simulink library "thc"  (R2021b)
settings: Solver=VariableStepAuto  StartTime=0.0  StopTime=10.0  RelTol=1e-3
undefined symbols (not defined in the file): ATHC_APTCQA_X_C, ATHC_APTCQB_X_C, ATHC_dAy_X_C, ATHC_Qeq_X_kmh, ATHC_VbaseC_X_C, ATHC_VbaseC_Y_W, ATHC_VbaseD_X_C, ATHC_VbaseH_X_C, FALSE, KTHC_ACMaxMinT_sec, KTHC_aDeice_K, KTHC_AGSDefLv_K, KTHC_AGSLv1_K, KTHC_AGSLv2_K, KTHC_AGSLv3_K, KTHC_AGSLv4_K, KTHC_AGSLv5_K, KTHC_AirIntUpdateT_sec, KTHC_APTCOneZoneMax_W, KTHC_APTCPeriod_cnt, KTHC_APTCPWMEN_flg, KTHC_APTCQMaxC_W, KTHC_APTCQminC_W, KTHC_APTCQminD_W, KTHC_APTCQminRe1_W, KTHC_APTCQminRe_W, KTHC_APTCQoffT_cnt, KTHC_APTCQonT_cnt, KTHC_APTCRiLeMaxDff_W, KTHC_APTCRiLeMinDff_W, KTHC_BatCoolT_cnt, KTHC_BatInTempDef_C, KTHC_bDeice_K, KTHC_CompMaxDeice_rpm, KTHC_CompMinDeice_rpm, KTHC_CompSotxvOp_K, KTHC_CompSotxvOpLow_rpm, KTHC_CompSpdmax_rpm, KTHC_CompSpdmaxBC1_rpm, KTHC_CompSpdmaxBC_rpm, KTHC_CompSpdmid1_rpm, KTHC_CompSpdmid2_rpm, KTHC_CompSpdmid3_rpm, KTHC_CompSpdmid_rpm, KTHC_CompSpdmin_rpm, KTHC_DAPTCQ1_W, KTHC_DAPTCQ2_W, KTHC_DAPTCQ3_W, KTHC_DcChSetTemp_C, KTHC_DehumidityEN_flg, KTHC_DeiceCycTime_K, KTHC_DriveLevelWPTCBAH1_W, KTHC_DriveLevelWPTCBAH2_W, KTHC_DriveLevelWPTCBAH3_W, KTHC_DriveLevelWPTCBAH4_W, KTHC_DriverSeatPos_flg, KTHC_DriveT1MinBAH_C, KTHC_DriveT2MaxBAH_C, KTHC_DriveT2MinBAH_C, KTHC_DriveT3MaxBAH_C ... (+379)
libraries: simulink x489
(part 10 of 17)

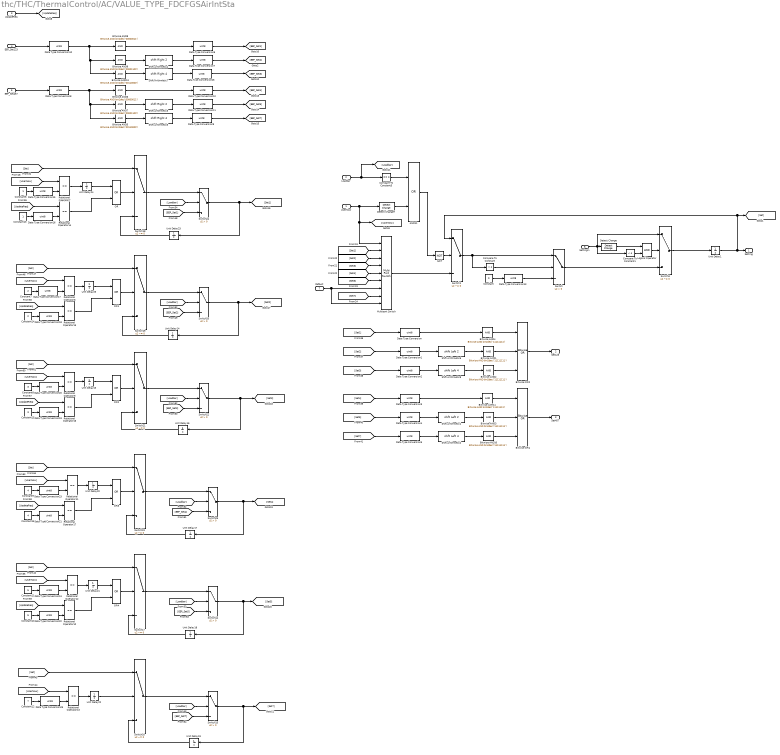
== system thc/THC/ThermalControl/AC/VALUE_TYPE_FDCFGSAirIntSta ==
  UserNow : Inport
  Loadbar : Inport  Port=2
  UpdateReq : Inport  Port=3
  EEP_Set123 : Inport  Port=4
  EEP_Set457 : Inport  Port=5
  SettingIn : Inport  Port=6
  Default : Inport  Port=7
  AND11 : Logic  Operator=OR  AllPortsSameDT=off  OutDataTypeStr=boolean
  Bitwise AND{1..4,10..11} (6 alike) : simulink/Logic and Bit Operations/Bitwise Operator  logicop=AND  UseBitMask=on  BitMask=bin2dec('11111111')  BitMaskRealWorld=Stored Integer
  Bitwise AND13 : simulink/Logic and Bit Operations/Bitwise Operator  logicop=AND  UseBitMask=on  BitMask=bin2dec('00110000')  BitMaskRealWorld=Stored Integer
  Bitwise AND5 : simulink/Logic and Bit Operations/Bitwise Operator  logicop=AND  UseBitMask=on  BitMask=bin2dec('00110000')  BitMaskRealWorld=Stored Integer
  Bitwise AND6 : simulink/Logic and Bit Operations/Bitwise Operator  logicop=AND  UseBitMask=on  BitMask=bin2dec('00000011')  BitMaskRealWorld=Stored Integer
  Bitwise AND7 : simulink/Logic and Bit Operations/Bitwise Operator  logicop=AND  UseBitMask=on  BitMask=bin2dec('00001100')  BitMaskRealWorld=Stored Integer
  Bitwise AND8 : simulink/Logic and Bit Operations/Bitwise Operator  logicop=AND  UseBitMask=on  BitMask=bin2dec('00000011')  BitMaskRealWorld=Stored Integer
  Bitwise AND9 : simulink/Logic and Bit Operations/Bitwise Operator  logicop=AND  UseBitMask=on  BitMask=bin2dec('00001100')  BitMaskRealWorld=Stored Integer
  Bitwise OR1 : simulink/Logic and Bit Operations/Bitwise Operator  logicop=OR  UseBitMask=off  NumInputPorts=3  BitMask=bin2dec('00000000000000000000')  BitMaskRealWorld=Stored Integer
  Bitwise OR2 : simulink/Logic and Bit Operations/Bitwise Operator  logicop=OR  UseBitMask=off  NumInputPorts=3  BitMask=bin2dec('00000000000000000000')  BitMaskRealWorld=Stored Integer
  Compare To Constant : simulink/Logic and Bit Operations/Compare To Constant  relop=<  const=4  OutDataTypeStr=boolean
  Compare To Constant1 : simulink/Logic and Bit Operations/Compare To Constant  relop=<  const=4  OutDataTypeStr=boolean
  Compare To Constant5 : simulink/Logic and Bit Operations/Compare To Constant  relop===  const=0  OutDataTypeStr=boolean
  Constant : Constant  Value=0
  Constant10 : Constant  Value=5  OutDataTypeStr=uint8
  Constant11 : Constant  Value=5  OutDataTypeStr=uint8
  Constant12 : Constant  Value=7  OutDataTypeStr=uint8
  Constant13 : Constant  OutDataTypeStr=uint8
  Constant14 : Constant  Value=2  OutDataTypeStr=uint8
  Constant15 : Constant  Value=3  OutDataTypeStr=uint8
  Constant16 : Constant  Value=4  OutDataTypeStr=uint8
  Constant6 : Constant  OutDataTypeStr=uint8
  Constant7 : Constant  Value=2  OutDataTypeStr=uint8
  Constant8 : Constant  Value=3  OutDataTypeStr=uint8
  Constant9 : Constant  Value=4  OutDataTypeStr=uint8
  Data Type Conversion{,1..13,15..26} (26 alike) : DataTypeConversion  OutDataTypeStr=uint8
  Detect Change : simulink/Logic and Bit Operations/Detect Change  vinit=0  OutDataTypeStr=boolean
  Detect Change7 : simulink/Logic and Bit Operations/Detect Change  vinit=0  OutDataTypeStr=boolean
  Logical Operator : Logic  AllPortsSameDT=off  OutDataTypeStr=boolean
  Multiport Switch : MultiPortSwitch  Inputs=7  DataPortForDefault=Additional data port  DiagnosticForDefault=None
  NOT : Logic  Operator=NOT  IconShape=distinctive  AllPortsSameDT=off  OutDataTypeStr=boolean
  OR{,1..4} (5 alike) : Logic  Operator=OR  AllPortsSameDT=off  OutDataTypeStr=boolean
  Relational Operator{7..17} (11 alike) : RelationalOperator  Operator===  OutDataTypeStr=boolean  RndMeth=Simplest
  Shift Arithmetic1 : ArithShift  BitShiftNumber=2  BitShiftDirection=Left
  Shift Arithmetic2 : ArithShift  BitShiftNumber=4  BitShiftDirection=Left
  Shift Arithmetic3 : ArithShift  BitShiftNumber=2  BitShiftDirection=Right
  Shift Arithmetic4 : ArithShift  BitShiftNumber=2  BitShiftDirection=Right
  Shift Arithmetic5 : ArithShift  BitShiftNumber=4  BitShiftDirection=Right
  Shift Arithmetic6 : ArithShift  BitShiftNumber=2  BitShiftDirection=Left
  Shift Arithmetic7 : ArithShift  BitShiftNumber=4  BitShiftDirection=Right
  Shift Arithmetic8 : ArithShift  BitShiftNumber=4  BitShiftDirection=Left
  Switch{,14..15,20,22,24..25} (7 alike) : Switch  Criteria=u2 > Threshold
  Switch{1,3,16..19,21,23} (8 alike) : Switch  Criteria=u2 ~= 0
  Unit Delay{1,14..25} (13 alike) : UnitDelay  SampleTime=-1  HasFrameUpgradeWarning=on
  Setting : Outport
  Set123 : Outport  Port=2
  Set457 : Outport  Port=3
  wires:
  Constant13/1 -> Data Type Conversion16/1
  Unit Delay19/1 -> Switch16/3
  Unit Delay23/1 -> Switch18/3
  OR2/1 -> Switch21/2
  Data Type Conversion20/1 -> Relational Operator9/2
  Unit Delay24/1 -> OR/1
  OR4/1 -> Switch17/2
  Relational Operator7/1 -> Unit Delay24/1
  Relational Operator14/1 -> OR/2
  [EEP_Set5] -> Switch14/3
  OR/1 -> Switch18/2
  [EEP_Set2] -> Switch20/3
  [UserNow] -> Relational Operator8/1
  Data Type Conversion15/1 -> Relational Operator7/2
  [EEP_Set3] -> Switch22/3
  Data Type Conversion19/1 -> Relational Operator16/2
  Unit Delay17/1 -> Switch23/3
  Constant16/1 -> Data Type Conversion21/1
  Constant15/1 -> Data Type Conversion19/1
  [UpdateReq] -> Relational Operator10/1
  [UpdateReq] -> Relational Operator17/1
  Switch22/1 -> [Set3], Unit Delay16/1
  Switch18/1 -> Switch24/1
  Unit Delay20/1 -> OR3/1
  Relational Operator17/1 -> OR3/2
  Data Type Conversion22/1 -> Relational Operator10/2
  Unit Delay15/1 -> OR2/1
  Constant11/1 -> Data Type Conversion24/1
  Data Type Conversion21/1 -> Relational Operator17/2
  Relational Operator16/1 -> OR2/2
  [UpdateReq] -> Relational Operator16/1
  Constant14/1 -> Data Type Conversion18/1
  Data Type Conversion17/1 -> Relational Operator8/2
  OR1/1 -> Switch19/2
  Data Type Conversion18/1 -> Relational Operator15/2
  Constant8/1 -> Data Type Conversion20/1
  [UpdateReq] -> Relational Operator15/1
  Unit Delay16/1 -> Switch21/3
  [Set] -> Switch16/1
  Data Type Conversion24/1 -> Relational Operator12/2
  [UserNow] -> Relational Operator12/1
  [Loadbar] -> Switch24/2
  Switch24/1 -> [Set1], Unit Delay23/1
  Unit Delay25/1 -> OR1/1
  Data Type Conversion16/1 -> Relational Operator14/2
  Relational Operator8/1 -> Unit Delay25/1
  [UserNow] -> Relational Operator9/1
  [Loadbar] -> Switch25/2
  [Set] -> Switch23/1
  [Set] -> Switch21/1
  [Loadbar] -> Switch15/2
  [UserNow] -> Relational Operator7/1
  Constant6/1 -> Data Type Conversion15/1
  [Loadbar] -> Switch22/2
  Data Type Conversion25/1 -> Relational Operator13/2
  Constant7/1 -> Data Type Conversion17/1
  [Set] -> Switch19/1
  OR3/1 -> Switch23/2
  [UserNow] -> Relational Operator13/1
  Switch25/1 -> [Set4], Unit Delay17/1
  Relational Operator11/1 -> Unit Delay20/1
  [Loadbar] -> Switch20/2
  [Set] -> Switch17/1
  Constant12/1 -> Data Type Conversion25/1
  Switch23/1 -> Switch25/1
  Unit Delay18/1 -> Switch17/3
  [UserNow] -> Relational Operator11/1
  [EEP_Set4] -> Switch25/3
  [Set] -> Switch18/1
  Constant9/1 -> Data Type Conversion23/1
  [EEP_Set7] -> Switch15/3
  Switch20/1 -> [Set2], Unit Delay14/1
  Unit Delay14/1 -> Switch19/3
  Switch17/1 -> Switch14/1
  Switch21/1 -> Switch22/1
  [EEP_Set1] -> Switch24/3
  [Loadbar] -> Switch14/2
  Relational Operator12/1 -> Unit Delay21/1
  [UpdateReq] -> Relational Operator14/1
  Switch19/1 -> Switch20/1
  Unit Delay22/1 -> Switch16/2
  Relational Operator9/1 -> Unit Delay15/1
  Relational Operator13/1 -> Unit Delay22/1
  Constant10/1 -> Data Type Conversion22/1
  Switch15/1 -> [Set7], Unit Delay19/1
  Switch16/1 -> Switch15/1
  Switch14/1 -> [Set5], Unit Delay18/1
  Relational Operator15/1 -> OR1/2
  Unit Delay21/1 -> OR4/1
  Data Type Conversion23/1 -> Relational Operator11/2
  Relational Operator10/1 -> OR4/2
  UpdateReq/1 -> [UpdateReq]
  Data Type Conversion12/1 -> Bitwise AND8/1, Bitwise AND13/1, Bitwise AND9/1
  EEP_Set123/1 -> Data Type Conversion12/1
  [Set3] -> Data Type Conversion2/1
  Data Type Conversion9/1 -> [EEP_Set7]
  Data Type Conversion11/1 -> [EEP_Set5]
  Data Type Conversion10/1 -> [EEP_Set4]
  Data Type Conversion7/1 -> [EEP_Set2]
  Data Type Conversion6/1 -> [EEP_Set1]
  Shift Arithmetic4/1 -> Data Type Conversion7/1
  Bitwise AND8/1 -> Data Type Conversion6/1
  Bitwise AND9/1 -> Shift Arithmetic4/1
  [Set2] -> Data Type Conversion1/1
  [Set1] -> Data Type Conversion/1
  Bitwise OR2/1 -> Set123/1
  Bitwise AND4/1 -> Bitwise OR2/1
  Data Type Conversion1/1 -> Shift Arithmetic6/1
  Bitwise AND1/1 -> Bitwise OR2/2
  Data Type Conversion2/1 -> Shift Arithmetic8/1
  Data Type Conversion/1 -> Bitwise AND4/1
  Shift Arithmetic6/1 -> Bitwise AND1/1
  Bitwise AND2/1 -> Bitwise OR2/3
  Unit Delay1/1 -> [Set], Switch1/1, Setting/1
  Switch3/1 -> Unit Delay1/1
  Loadbar/1 -> Compare To Constant5/1, [Loadbar]
  UserNow/1 -> Detect Change7/1, [UserNow], Multiport Switch/1
  Compare To Constant5/1 -> AND11/1
  AND11/1 -> NOT/1
  Switch/1 -> Switch3/3
  Multiport Switch/1 -> Switch1/3
  Detect Change7/1 -> AND11/2
  NOT/1 -> Switch1/2
  [Set1] -> Multiport Switch/2
  [Set2] -> Multiport Switch/3
  [Set3] -> Multiport Switch/4
  [Set4] -> Multiport Switch/5
  [Set5] -> Multiport Switch/6
  [Set7] -> Multiport Switch/8
  Default/1 -> Multiport Switch/9, Multiport Switch/7
  SettingIn/1 -> Compare To Constant1/1, Switch3/1, Detect Change/1
  Bitwise AND13/1 -> Shift Arithmetic7/1
  Shift Arithmetic7/1 -> Data Type Conversion26/1
  Data Type Conversion26/1 -> [EEP_Set3]
  Shift Arithmetic8/1 -> Bitwise AND2/1
  Detect Change/1 -> Logical Operator/1
  Shift Arithmetic5/1 -> Data Type Conversion9/1
  Bitwise AND5/1 -> Shift Arithmetic5/1
  Bitwise AND7/1 -> Shift Arithmetic3/1
  Bitwise AND6/1 -> Data Type Conversion10/1
  Shift Arithmetic3/1 -> Data Type Conversion11/1
  EEP_Set457/1 -> Data Type Conversion8/1
  Data Type Conversion8/1 -> Bitwise AND7/1, Bitwise AND5/1, Bitwise AND6/1
  Shift Arithmetic2/1 -> Bitwise AND10/1
  Bitwise AND10/1 -> Bitwise OR1/3
  Shift Arithmetic1/1 -> Bitwise AND3/1
  Data Type Conversion3/1 -> Bitwise AND11/1
  Data Type Conversion5/1 -> Shift Arithmetic2/1
  Bitwise AND3/1 -> Bitwise OR1/2
  Data Type Conversion4/1 -> Shift Arithmetic1/1
  Bitwise AND11/1 -> Bitwise OR1/1
  [Set4] -> Data Type Conversion3/1
  [Set5] -> Data Type Conversion4/1
  [Set7] -> Data Type Conversion5/1
  Bitwise OR1/1 -> Set457/1
  Switch1/1 -> Compare To Constant/1, Switch/1
  Compare To Constant/1 -> Switch/2
  Constant/1 -> Data Type Conversion13/1
  Data Type Conversion13/1 -> Switch/3
  Compare To Constant1/1 -> Logical Operator/2
  Logical Operator/1 -> Switch3/2

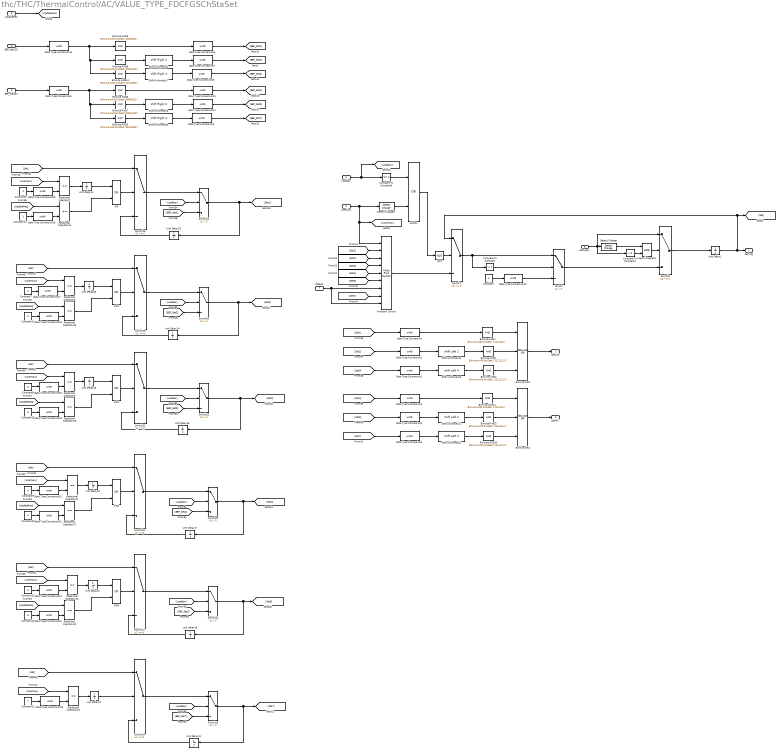
== system thc/THC/ThermalControl/AC/VALUE_TYPE_FDCFGSChStaSet ==
  UserNow : Inport
  Loadbar : Inport  Port=2
  UpdateReq : Inport  Port=3
  EEP_Set123 : Inport  Port=4
  EEP_Set457 : Inport  Port=5
  SettingIn : Inport  Port=6
  Default : Inport  Port=7
  AND11 : Logic  Operator=OR  AllPortsSameDT=off  OutDataTypeStr=boolean
  Bitwise AND{1..4,10..11} (6 alike) : simulink/Logic and Bit Operations/Bitwise Operator  logicop=AND  UseBitMask=on  BitMask=bin2dec('11111111')  BitMaskRealWorld=Stored Integer
  Bitwise AND13 : simulink/Logic and Bit Operations/Bitwise Operator  logicop=AND  UseBitMask=on  BitMask=bin2dec('00110000')  BitMaskRealWorld=Stored Integer
  Bitwise AND5 : simulink/Logic and Bit Operations/Bitwise Operator  logicop=AND  UseBitMask=on  BitMask=bin2dec('00110000')  BitMaskRealWorld=Stored Integer
  Bitwise AND6 : simulink/Logic and Bit Operations/Bitwise Operator  logicop=AND  UseBitMask=on  BitMask=bin2dec('00000011')  BitMaskRealWorld=Stored Integer
  Bitwise AND7 : simulink/Logic and Bit Operations/Bitwise Operator  logicop=AND  UseBitMask=on  BitMask=bin2dec('00001100')  BitMaskRealWorld=Stored Integer
  Bitwise AND8 : simulink/Logic and Bit Operations/Bitwise Operator  logicop=AND  UseBitMask=on  BitMask=bin2dec('00000011')  BitMaskRealWorld=Stored Integer
  Bitwise AND9 : simulink/Logic and Bit Operations/Bitwise Operator  logicop=AND  UseBitMask=on  BitMask=bin2dec('00001100')  BitMaskRealWorld=Stored Integer
  Bitwise OR1 : simulink/Logic and Bit Operations/Bitwise Operator  logicop=OR  UseBitMask=off  NumInputPorts=3  BitMask=bin2dec('00000000000000000000')  BitMaskRealWorld=Stored Integer
  Bitwise OR2 : simulink/Logic and Bit Operations/Bitwise Operator  logicop=OR  UseBitMask=off  NumInputPorts=3  BitMask=bin2dec('00000000000000000000')  BitMaskRealWorld=Stored Integer
  Compare To Constant : simulink/Logic and Bit Operations/Compare To Constant  relop=>  const=0  OutDataTypeStr=boolean
  Compare To Constant1 : simulink/Logic and Bit Operations/Compare To Constant  relop=>  const=0  OutDataTypeStr=boolean
  Compare To Constant5 : simulink/Logic and Bit Operations/Compare To Constant  relop===  const=0  OutDataTypeStr=boolean
  Constant : Constant
  Constant10 : Constant  Value=5  OutDataTypeStr=uint8
  Constant11 : Constant  Value=5  OutDataTypeStr=uint8
  Constant12 : Constant  Value=7  OutDataTypeStr=uint8
  Constant13 : Constant  OutDataTypeStr=uint8
  Constant14 : Constant  Value=2  OutDataTypeStr=uint8
  Constant15 : Constant  Value=3  OutDataTypeStr=uint8
  Constant16 : Constant  Value=4  OutDataTypeStr=uint8
  Constant6 : Constant  OutDataTypeStr=uint8
  Constant7 : Constant  Value=2  OutDataTypeStr=uint8
  Constant8 : Constant  Value=3  OutDataTypeStr=uint8
  Constant9 : Constant  Value=4  OutDataTypeStr=uint8
  Data Type Conversion{,1..13,15..26} (26 alike) : DataTypeConversion  OutDataTypeStr=uint8
  Detect Change : simulink/Logic and Bit Operations/Detect Change  vinit=0  OutDataTypeStr=boolean
  Detect Change7 : simulink/Logic and Bit Operations/Detect Change  vinit=0  OutDataTypeStr=boolean
  Logical Operator : Logic  AllPortsSameDT=off  OutDataTypeStr=boolean
  Multiport Switch : MultiPortSwitch  Inputs=7  DataPortForDefault=Additional data port  DiagnosticForDefault=None
  NOT : Logic  Operator=NOT  IconShape=distinctive  AllPortsSameDT=off  OutDataTypeStr=boolean
  OR{,1..4} (5 alike) : Logic  Operator=OR  AllPortsSameDT=off  OutDataTypeStr=boolean
  Relational Operator{7..17} (11 alike) : RelationalOperator  Operator===  OutDataTypeStr=boolean  RndMeth=Simplest
  Shift Arithmetic1 : ArithShift  BitShiftNumber=2  BitShiftDirection=Left
  Shift Arithmetic2 : ArithShift  BitShiftNumber=4  BitShiftDirection=Left
  Shift Arithmetic3 : ArithShift  BitShiftNumber=2  BitShiftDirection=Right
  Shift Arithmetic4 : ArithShift  BitShiftNumber=2  BitShiftDirection=Right
  Shift Arithmetic5 : ArithShift  BitShiftNumber=4  BitShiftDirection=Right
  Shift Arithmetic6 : ArithShift  BitShiftNumber=2  BitShiftDirection=Left
  Shift Arithmetic7 : ArithShift  BitShiftNumber=4  BitShiftDirection=Right
  Shift Arithmetic8 : ArithShift  BitShiftNumber=4  BitShiftDirection=Left
  Switch{,14..15,20,22,24..25} (7 alike) : Switch  Criteria=u2 > Threshold
  Switch{1,3,16..19,21,23} (8 alike) : Switch  Criteria=u2 ~= 0
  Unit Delay{1,14..25} (13 alike) : UnitDelay  SampleTime=-1  HasFrameUpgradeWarning=on
  Setting : Outport
  Set123 : Outport  Port=2
  Set457 : Outport  Port=3
  wires:
  Logical Operator/1 -> Switch3/2
  Compare To Constant1/1 -> Logical Operator/2
  Data Type Conversion13/1 -> Switch/3
  Constant/1 -> Data Type Conversion13/1
  Compare To Constant/1 -> Switch/2
  Switch1/1 -> Switch/1, Compare To Constant/1
  Bitwise OR1/1 -> Set457/1
  [Set7] -> Data Type Conversion5/1
  [Set5] -> Data Type Conversion4/1
  [Set4] -> Data Type Conversion3/1
  Bitwise AND11/1 -> Bitwise OR1/1
  Data Type Conversion4/1 -> Shift Arithmetic1/1
  Bitwise AND3/1 -> Bitwise OR1/2
  Data Type Conversion5/1 -> Shift Arithmetic2/1
  Data Type Conversion3/1 -> Bitwise AND11/1
  Shift Arithmetic1/1 -> Bitwise AND3/1
  Bitwise AND10/1 -> Bitwise OR1/3
  Shift Arithmetic2/1 -> Bitwise AND10/1
  Data Type Conversion8/1 -> Bitwise AND6/1, Bitwise AND5/1, Bitwise AND7/1
  EEP_Set457/1 -> Data Type Conversion8/1
  Shift Arithmetic3/1 -> Data Type Conversion11/1
  Bitwise AND6/1 -> Data Type Conversion10/1
  Bitwise AND7/1 -> Shift Arithmetic3/1
  Bitwise AND5/1 -> Shift Arithmetic5/1
  Shift Arithmetic5/1 -> Data Type Conversion9/1
  Detect Change/1 -> Logical Operator/1
  Shift Arithmetic8/1 -> Bitwise AND2/1
  Data Type Conversion26/1 -> [EEP_Set3]
  Shift Arithmetic7/1 -> Data Type Conversion26/1
  Bitwise AND13/1 -> Shift Arithmetic7/1
  SettingIn/1 -> Detect Change/1, Switch3/1, Compare To Constant1/1
  Default/1 -> Multiport Switch/7, Multiport Switch/9
  [Set7] -> Multiport Switch/8
  [Set5] -> Multiport Switch/6
  [Set4] -> Multiport Switch/5
  [Set3] -> Multiport Switch/4
  [Set2] -> Multiport Switch/3
  [Set1] -> Multiport Switch/2
  NOT/1 -> Switch1/2
  Detect Change7/1 -> AND11/2
  Multiport Switch/1 -> Switch1/3
  Switch/1 -> Switch3/3
  AND11/1 -> NOT/1
  Compare To Constant5/1 -> AND11/1
  UserNow/1 -> Multiport Switch/1, [UserNow], Detect Change7/1
  Loadbar/1 -> [Loadbar], Compare To Constant5/1
  Switch3/1 -> Unit Delay1/1
  Unit Delay1/1 -> Setting/1, Switch1/1, [Set]
  Bitwise AND2/1 -> Bitwise OR2/3
  Shift Arithmetic6/1 -> Bitwise AND1/1
  Data Type Conversion/1 -> Bitwise AND4/1
  Data Type Conversion2/1 -> Shift Arithmetic8/1
  Bitwise AND1/1 -> Bitwise OR2/2
  Data Type Conversion1/1 -> Shift Arithmetic6/1
  Bitwise AND4/1 -> Bitwise OR2/1
  Bitwise OR2/1 -> Set123/1
  [Set1] -> Data Type Conversion/1
  [Set2] -> Data Type Conversion1/1
  Bitwise AND9/1 -> Shift Arithmetic4/1
  Bitwise AND8/1 -> Data Type Conversion6/1
  Shift Arithmetic4/1 -> Data Type Conversion7/1
  Data Type Conversion6/1 -> [EEP_Set1]
  Data Type Conversion7/1 -> [EEP_Set2]
  Data Type Conversion10/1 -> [EEP_Set4]
  Data Type Conversion11/1 -> [EEP_Set5]
  Data Type Conversion9/1 -> [EEP_Set7]
  [Set3] -> Data Type Conversion2/1
  EEP_Set123/1 -> Data Type Conversion12/1
  Data Type Conversion12/1 -> Bitwise AND9/1, Bitwise AND13/1, Bitwise AND8/1
  UpdateReq/1 -> [UpdateReq]
  Relational Operator10/1 -> OR4/2
  Data Type Conversion23/1 -> Relational Operator11/2
  Unit Delay21/1 -> OR4/1
  Relational Operator15/1 -> OR1/2
  Switch14/1 -> Unit Delay18/1, [Set5]
  Switch16/1 -> Switch15/1
  Switch15/1 -> Unit Delay19/1, [Set7]
  Constant10/1 -> Data Type Conversion22/1
  Relational Operator13/1 -> Unit Delay22/1
  Relational Operator9/1 -> Unit Delay15/1
  Unit Delay22/1 -> Switch16/2
  Switch19/1 -> Switch20/1
  [UpdateReq] -> Relational Operator14/1
  Relational Operator12/1 -> Unit Delay21/1
  [Loadbar] -> Switch14/2
  [EEP_Set1] -> Switch24/3
  Switch21/1 -> Switch22/1
  Switch17/1 -> Switch14/1
  Unit Delay14/1 -> Switch19/3
  Switch20/1 -> Unit Delay14/1, [Set2]
  [EEP_Set7] -> Switch15/3
  Constant9/1 -> Data Type Conversion23/1
  [Set] -> Switch18/1
  [EEP_Set4] -> Switch25/3
  [UserNow] -> Relational Operator11/1
  Unit Delay18/1 -> Switch17/3
  Switch23/1 -> Switch25/1
  Constant12/1 -> Data Type Conversion25/1
  [Set] -> Switch17/1
  [Loadbar] -> Switch20/2
  Relational Operator11/1 -> Unit Delay20/1
  Switch25/1 -> Unit Delay17/1, [Set4]
  [UserNow] -> Relational Operator13/1
  OR3/1 -> Switch23/2
  [Set] -> Switch19/1
  Constant7/1 -> Data Type Conversion17/1
  Data Type Conversion25/1 -> Relational Operator13/2
  [Loadbar] -> Switch22/2
  Constant6/1 -> Data Type Conversion15/1
  [UserNow] -> Relational Operator7/1
  [Loadbar] -> Switch15/2
  [Set] -> Switch21/1
  [Set] -> Switch23/1
  [Loadbar] -> Switch25/2
  [UserNow] -> Relational Operator9/1
  Relational Operator8/1 -> Unit Delay25/1
  Data Type Conversion16/1 -> Relational Operator14/2
  Unit Delay25/1 -> OR1/1
  Switch24/1 -> Unit Delay23/1, [Set1]
  [Loadbar] -> Switch24/2
  [UserNow] -> Relational Operator12/1
  Data Type Conversion24/1 -> Relational Operator12/2
  [Set] -> Switch16/1
  Unit Delay16/1 -> Switch21/3
  [UpdateReq] -> Relational Operator15/1
  Constant8/1 -> Data Type Conversion20/1
  Data Type Conversion18/1 -> Relational Operator15/2
  OR1/1 -> Switch19/2
  Data Type Conversion17/1 -> Relational Operator8/2
  Constant14/1 -> Data Type Conversion18/1
  [UpdateReq] -> Relational Operator16/1
  Relational Operator16/1 -> OR2/2
  Data Type Conversion21/1 -> Relational Operator17/2
  Constant11/1 -> Data Type Conversion24/1
  Unit Delay15/1 -> OR2/1
  Data Type Conversion22/1 -> Relational Operator10/2
  Relational Operator17/1 -> OR3/2
  Unit Delay20/1 -> OR3/1
  Switch18/1 -> Switch24/1
  Switch22/1 -> Unit Delay16/1, [Set3]
  [UpdateReq] -> Relational Operator17/1
  [UpdateReq] -> Relational Operator10/1
  Constant15/1 -> Data Type Conversion19/1
  Constant16/1 -> Data Type Conversion21/1
  Unit Delay17/1 -> Switch23/3
  Data Type Conversion19/1 -> Relational Operator16/2
  [EEP_Set3] -> Switch22/3
  Data Type Conversion15/1 -> Relational Operator7/2
  [UserNow] -> Relational Operator8/1
  [EEP_Set2] -> Switch20/3
  OR/1 -> Switch18/2
  [EEP_Set5] -> Switch14/3
  Relational Operator14/1 -> OR/2
  Relational Operator7/1 -> Unit Delay24/1
  OR4/1 -> Switch17/2
  Unit Delay24/1 -> OR/1
  Data Type Conversion20/1 -> Relational Operator9/2
  OR2/1 -> Switch21/2
  Unit Delay23/1 -> Switch18/3
  Unit Delay19/1 -> Switch16/3
  Constant13/1 -> Data Type Conversion16/1

== system thc/THC/ThermalControl/AC/VALUE_TYPE_FDCTHCCLEVentYSta ==
  UserNow : Inport
  Loadbar : Inport  Port=2
  UpdateReq : Inport  Port=3
  SettingIN : Inport  Port=4
  EEP_Set1 : Inport  Port=5
  EEP_Set2 : Inport  Port=6
  EEP_Set3 : Inport  Port=7
  EEP_Set4 : Inport  Port=8
  EEP_Set5 : Inport  Port=9
  EEP_Set7 : Inport  Port=10
  Default : Inport  Port=11
  AND11 : Logic  Operator=OR  AllPortsSameDT=off  OutDataTypeStr=boolean
  Compare To Constant5 : simulink/Logic and Bit Operations/Compare To Constant  relop===  const=0  OutDataTypeStr=boolean
  Constant : Constant  OutDataTypeStr=uint8
  Constant1 : Constant  Value=2  OutDataTypeStr=uint8
  Constant10 : Constant  Value=5  OutDataTypeStr=uint8
  Constant2 : Constant  Value=3  OutDataTypeStr=uint8
  Constant3 : Constant  Value=4  OutDataTypeStr=uint8
  Constant4 : Constant  Value=5  OutDataTypeStr=uint8
  Constant5 : Constant  Value=7  OutDataTypeStr=uint8
  Constant6 : Constant  OutDataTypeStr=uint8
  Constant7 : Constant  Value=2  OutDataTypeStr=uint8
  Constant8 : Constant  Value=3  OutDataTypeStr=uint8
  Constant9 : Constant  Value=4  OutDataTypeStr=uint8
  Data Type Conversion{1..9,13} (10 alike) : DataTypeConversion  OutDataTypeStr=uint8
  Detect Change1 : simulink/Logic and Bit Operations/Detect Change  vinit=0  OutDataTypeStr=boolean
  Detect Change7 : simulink/Logic and Bit Operations/Detect Change  vinit=0  OutDataTypeStr=boolean
  Logical Operator1 : Logic  AllPortsSameDT=off  OutDataTypeStr=boolean
  Multiport Switch : MultiPortSwitch  Inputs=7  DataPortForDefault=Additional data port  DiagnosticForDefault=None
  NOT : Logic  Operator=NOT  IconShape=distinctive  AllPortsSameDT=off  OutDataTypeStr=boolean
  OR{,1..4} (5 alike) : Logic  Operator=OR  AllPortsSameDT=off  OutDataTypeStr=boolean
  Relational Operator{,1..5,7..11} (11 alike) : RelationalOperator  Operator===  OutDataTypeStr=boolean  RndMeth=Simplest
  Switch{,1..3,5,7..8,12..13} (9 alike) : Switch  Criteria=u2 ~= 0
  Switch{4,6,9..11} (5 alike) : Switch  Criteria=u2 > Threshold
  Unit Delay{1..13} (13 alike) : UnitDelay  SampleTime=-1  HasFrameUpgradeWarning=on
  Setting : Outport
  Set1 : Outport  Port=2
  Set2 : Outport  Port=3
  Set3 : Outport  Port=4
  Set4 : Outport  Port=5
  Set5 : Outport  Port=6
  Set7 : Outport  Port=7
  wires:
  [Loadbar] -> Logical Operator1/2
  Data Type Conversion9/1 -> Relational Operator4/2
  Unit Delay12/1 -> OR4/1
  OR4/1 -> Switch13/2
  Constant10/1 -> Data Type Conversion8/1
  [UpdateReq] -> Relational Operator11/1
  Data Type Conversion8/1 -> Relational Operator11/2
  Relational Operator11/1 -> OR4/2
  Data Type Conversion7/1 -> Relational Operator3/2
  Constant3/1 -> Data Type Conversion7/1
  OR3/1 -> Switch7/2
  Unit Delay11/1 -> OR3/1
  Relational Operator10/1 -> OR3/2
  Data Type Conversion6/1 -> Relational Operator10/2
  [UpdateReq] -> Relational Operator10/1
  Constant9/1 -> Data Type Conversion6/1
  Data Type Conversion5/1 -> Relational Operator2/2
  Constant2/1 -> Data Type Conversion5/1
  OR2/1 -> Switch5/2
  Unit Delay10/1 -> OR2/1
  Constant8/1 -> Data Type Conversion4/1
  [UpdateReq] -> Relational Operator9/1
  Data Type Conversion4/1 -> Relational Operator9/2
  Relational Operator9/1 -> OR2/2
  Data Type Conversion3/1 -> Relational Operator1/2
  Unit Delay9/1 -> OR1/1
  OR1/1 -> Switch3/2
  Relational Operator8/1 -> OR1/2
  Data Type Conversion2/1 -> Relational Operator8/2
  [UpdateReq] -> Relational Operator8/1
  Constant7/1 -> Data Type Conversion2/1
  Data Type Conversion1/1 -> Relational Operator/2
  Unit Delay6/1 -> OR/1
  OR/1 -> Switch2/2
  Constant6/1 -> Data Type Conversion13/1
  [UpdateReq] -> Relational Operator7/1
  Data Type Conversion13/1 -> Relational Operator7/2
  Relational Operator7/1 -> OR/2
  UpdateReq/1 -> [UpdateReq]
  Unit Delay13/1 -> Switch12/2
  Unit Delay5/1 -> Switch12/3
  Unit Delay4/1 -> Switch13/3
  Unit Delay3/1 -> Switch7/3
  Unit Delay8/1 -> Switch5/3
  Unit Delay2/1 -> Switch3/3
  Unit Delay7/1 -> Switch2/3
  Unit Delay1/1 -> Setting/1, [Set], Switch1/1
  Switch/1 -> Unit Delay1/1
  Loadbar/1 -> Compare To Constant5/1, [Loadbar]
  UserNow/1 -> Detect Change7/1, [UserNow], Multiport Switch/1
  Compare To Constant5/1 -> AND11/1
  AND11/1 -> NOT/1
  [Set7] -> Set7/1
  [Set5] -> Set5/1
  [Set4] -> Set4/1
  [Set3] -> Set3/1
  [Set2] -> Set2/1
  [Set1] -> Set1/1
  Switch1/1 -> Switch/3
  Logical Operator1/1 -> Switch/2
  Multiport Switch/1 -> Switch1/3
  SettingIN/1 -> Switch/1, Detect Change1/1
  Detect Change1/1 -> Logical Operator1/1
  Switch6/1 -> Unit Delay8/1, [Set3]
  Switch2/1 -> Switch8/1
  Switch12/1 -> Switch11/1
  Switch5/1 -> Switch6/1
  Switch13/1 -> Switch10/1
  [Set] -> Switch5/1
  EEP_Set1/1 -> Switch8/3
  Switch9/1 -> Unit Delay3/1, [Set4]
  EEP_Set7/1 -> Switch11/3
  [Loadbar] -> Switch9/2
  [Set] -> Switch12/1
  Relational Operator/1 -> Unit Delay6/1
  [Set] -> Switch13/1
  [Set] -> Switch3/1
  [Loadbar] -> Switch10/2
  Constant/1 -> Data Type Conversion1/1
  [Loadbar] -> Switch6/2
  [Loadbar] -> Switch11/2
  EEP_Set5/1 -> Switch10/3
  EEP_Set2/1 -> Switch4/3
  [UserNow] -> Relational Operator/1
  Switch4/1 -> Unit Delay2/1, [Set2]
  [Loadbar] -> Switch4/2
  [Set] -> Switch7/1
  EEP_Set4/1 -> Switch9/3
  Switch11/1 -> Unit Delay5/1, [Set7]
  EEP_Set3/1 -> Switch6/3
  [Loadbar] -> Switch8/2
  [UserNow] -> Relational Operator1/1
  Constant1/1 -> Data Type Conversion3/1
  Relational Operator1/1 -> Unit Delay9/1
  [UserNow] -> Relational Operator2/1
  Relational Operator2/1 -> Unit Delay10/1
  [UserNow] -> Relational Operator3/1
  Relational Operator3/1 -> Unit Delay11/1
  [UserNow] -> Relational Operator4/1
  Constant4/1 -> Data Type Conversion9/1
  Relational Operator4/1 -> Unit Delay12/1
  [UserNow] -> Relational Operator5/1
  Constant5/1 -> Relational Operator5/2
  Relational Operator5/1 -> Unit Delay13/1
  Switch3/1 -> Switch4/1
  Detect Change7/1 -> AND11/2
  Switch7/1 -> Switch9/1
  Switch10/1 -> Unit Delay4/1, [Set5]
  Switch8/1 -> Unit Delay7/1, [Set1]
  NOT/1 -> Switch1/2
  [Set] -> Switch2/1
  [Set1] -> Multiport Switch/2
  [Set2] -> Multiport Switch/3
  [Set3] -> Multiport Switch/4
  [Set4] -> Multiport Switch/5
  [Set5] -> Multiport Switch/6
  [Set7] -> Multiport Switch/8
  Default/1 -> Multiport Switch/9, Multiport Switch/7

== system thc/THC/ThermalControl/AC/VALUE_TYPE_FDCTHCCLEVentZSta ==
  UserNow : Inport
  Loadbar : Inport  Port=2
  UpdateReq : Inport  Port=3
  SettingIN : Inport  Port=4
  EEP_Set1 : Inport  Port=5
  EEP_Set2 : Inport  Port=6
  EEP_Set3 : Inport  Port=7
  EEP_Set4 : Inport  Port=8
  EEP_Set5 : Inport  Port=9
  EEP_Set7 : Inport  Port=10
  Default : Inport  Port=11
  AND11 : Logic  Operator=OR  AllPortsSameDT=off  OutDataTypeStr=boolean
  Compare To Constant5 : simulink/Logic and Bit Operations/Compare To Constant  relop===  const=0  OutDataTypeStr=boolean
  Constant : Constant  OutDataTypeStr=uint8
  Constant1 : Constant  Value=2  OutDataTypeStr=uint8
  Constant10 : Constant  Value=5  OutDataTypeStr=uint8
  Constant2 : Constant  Value=3  OutDataTypeStr=uint8
  Constant3 : Constant  Value=4  OutDataTypeStr=uint8
  Constant4 : Constant  Value=5  OutDataTypeStr=uint8
  Constant5 : Constant  Value=7  OutDataTypeStr=uint8
  Constant6 : Constant  OutDataTypeStr=uint8
  Constant7 : Constant  Value=2  OutDataTypeStr=uint8
  Constant8 : Constant  Value=3  OutDataTypeStr=uint8
  Constant9 : Constant  Value=4  OutDataTypeStr=uint8
  Data Type Conversion{1..9,13} (10 alike) : DataTypeConversion  OutDataTypeStr=uint8
  Detect Change1 : simulink/Logic and Bit Operations/Detect Change  vinit=0  OutDataTypeStr=boolean
  Detect Change7 : simulink/Logic and Bit Operations/Detect Change  vinit=0  OutDataTypeStr=boolean
  Logical Operator1 : Logic  AllPortsSameDT=off  OutDataTypeStr=boolean
  Multiport Switch : MultiPortSwitch  Inputs=7  DataPortForDefault=Additional data port  DiagnosticForDefault=None
  NOT : Logic  Operator=NOT  IconShape=distinctive  AllPortsSameDT=off  OutDataTypeStr=boolean
  OR{,1..4} (5 alike) : Logic  Operator=OR  AllPortsSameDT=off  OutDataTypeStr=boolean
  Relational Operator{,1..5,7..11} (11 alike) : RelationalOperator  Operator===  OutDataTypeStr=boolean  RndMeth=Simplest
  Switch{,1..3,5,7..8,12..13} (9 alike) : Switch  Criteria=u2 ~= 0
  Switch{4,6,9..11} (5 alike) : Switch  Criteria=u2 > Threshold
  Unit Delay{1..13} (13 alike) : UnitDelay  SampleTime=-1  HasFrameUpgradeWarning=on
  Setting : Outport
  Set1 : Outport  Port=2
  Set2 : Outport  Port=3
  Set3 : Outport  Port=4
  Set4 : Outport  Port=5
  Set5 : Outport  Port=6
  Set7 : Outport  Port=7
  wires:
  [Loadbar] -> Logical Operator1/2
  Data Type Conversion9/1 -> Relational Operator4/2
  Unit Delay12/1 -> OR4/1
  OR4/1 -> Switch13/2
  Constant10/1 -> Data Type Conversion8/1
  [UpdateReq] -> Relational Operator11/1
  Data Type Conversion8/1 -> Relational Operator11/2
  Relational Operator11/1 -> OR4/2
  Data Type Conversion7/1 -> Relational Operator3/2
  Constant3/1 -> Data Type Conversion7/1
  OR3/1 -> Switch7/2
  Unit Delay11/1 -> OR3/1
  Relational Operator10/1 -> OR3/2
  Data Type Conversion6/1 -> Relational Operator10/2
  [UpdateReq] -> Relational Operator10/1
  Constant9/1 -> Data Type Conversion6/1
  Data Type Conversion5/1 -> Relational Operator2/2
  Constant2/1 -> Data Type Conversion5/1
  OR2/1 -> Switch5/2
  Unit Delay10/1 -> OR2/1
  Constant8/1 -> Data Type Conversion4/1
  [UpdateReq] -> Relational Operator9/1
  Data Type Conversion4/1 -> Relational Operator9/2
  Relational Operator9/1 -> OR2/2
  Data Type Conversion3/1 -> Relational Operator1/2
  Unit Delay9/1 -> OR1/1
  OR1/1 -> Switch3/2
  Relational Operator8/1 -> OR1/2
  Data Type Conversion2/1 -> Relational Operator8/2
  [UpdateReq] -> Relational Operator8/1
  Constant7/1 -> Data Type Conversion2/1
  Data Type Conversion1/1 -> Relational Operator/2
  Unit Delay6/1 -> OR/1
  OR/1 -> Switch2/2
  Constant6/1 -> Data Type Conversion13/1
  [UpdateReq] -> Relational Operator7/1
  Data Type Conversion13/1 -> Relational Operator7/2
  Relational Operator7/1 -> OR/2
  UpdateReq/1 -> [UpdateReq]
  Unit Delay13/1 -> Switch12/2
  Unit Delay5/1 -> Switch12/3
  Unit Delay4/1 -> Switch13/3
  Unit Delay3/1 -> Switch7/3
  Unit Delay8/1 -> Switch5/3
  Unit Delay2/1 -> Switch3/3
  Unit Delay7/1 -> Switch2/3
  Unit Delay1/1 -> Setting/1, [Set], Switch1/1
  Switch/1 -> Unit Delay1/1
  Loadbar/1 -> Compare To Constant5/1, [Loadbar]
  UserNow/1 -> Detect Change7/1, [UserNow], Multiport Switch/1
  Compare To Constant5/1 -> AND11/1
  AND11/1 -> NOT/1
  [Set7] -> Set7/1
  [Set5] -> Set5/1
  [Set4] -> Set4/1
  [Set3] -> Set3/1
  [Set2] -> Set2/1
  [Set1] -> Set1/1
  Switch1/1 -> Switch/3
  Logical Operator1/1 -> Switch/2
  Multiport Switch/1 -> Switch1/3
  SettingIN/1 -> Switch/1, Detect Change1/1
  Detect Change1/1 -> Logical Operator1/1
  Switch6/1 -> Unit Delay8/1, [Set3]
  Switch2/1 -> Switch8/1
  Switch12/1 -> Switch11/1
  Switch5/1 -> Switch6/1
  Switch13/1 -> Switch10/1
  [Set] -> Switch5/1
  EEP_Set1/1 -> Switch8/3
  Switch9/1 -> Unit Delay3/1, [Set4]
  EEP_Set7/1 -> Switch11/3
  [Loadbar] -> Switch9/2
  [Set] -> Switch12/1
  Relational Operator/1 -> Unit Delay6/1
  [Set] -> Switch13/1
  [Set] -> Switch3/1
  [Loadbar] -> Switch10/2
  Constant/1 -> Data Type Conversion1/1
  [Loadbar] -> Switch6/2
  [Loadbar] -> Switch11/2
  EEP_Set5/1 -> Switch10/3
  EEP_Set2/1 -> Switch4/3
  [UserNow] -> Relational Operator/1
  Switch4/1 -> Unit Delay2/1, [Set2]
  [Loadbar] -> Switch4/2
  [Set] -> Switch7/1
  EEP_Set4/1 -> Switch9/3
  Switch11/1 -> Unit Delay5/1, [Set7]
  EEP_Set3/1 -> Switch6/3
  [Loadbar] -> Switch8/2
  [UserNow] -> Relational Operator1/1
  Constant1/1 -> Data Type Conversion3/1
  Relational Operator1/1 -> Unit Delay9/1
  [UserNow] -> Relational Operator2/1
  Relational Operator2/1 -> Unit Delay10/1
  [UserNow] -> Relational Operator3/1
  Relational Operator3/1 -> Unit Delay11/1
  [UserNow] -> Relational Operator4/1
  Constant4/1 -> Data Type Conversion9/1
  Relational Operator4/1 -> Unit Delay12/1
  [UserNow] -> Relational Operator5/1
  Constant5/1 -> Relational Operator5/2
  Relational Operator5/1 -> Unit Delay13/1
  Switch3/1 -> Switch4/1
  Detect Change7/1 -> AND11/2
  Switch7/1 -> Switch9/1
  Switch10/1 -> Unit Delay4/1, [Set5]
  Switch8/1 -> Unit Delay7/1, [Set1]
  NOT/1 -> Switch1/2
  [Set] -> Switch2/1
  [Set1] -> Multiport Switch/2
  [Set2] -> Multiport Switch/3
  [Set3] -> Multiport Switch/4
  [Set4] -> Multiport Switch/5
  [Set5] -> Multiport Switch/6
  [Set7] -> Multiport Switch/8
  Default/1 -> Multiport Switch/9, Multiport Switch/7

== system thc/THC/ThermalControl/AC/VALUE_TYPE_FDCTHCCREVentYSta ==
  UserNow : Inport
  Loadbar : Inport  Port=2
  UpdateReq : Inport  Port=3
  SettingIN : Inport  Port=4
  EEP_Set1 : Inport  Port=5
  EEP_Set2 : Inport  Port=6
  EEP_Set3 : Inport  Port=7
  EEP_Set4 : Inport  Port=8
  EEP_Set5 : Inport  Port=9
  EEP_Set7 : Inport  Port=10
  Default : Inport  Port=11
  AND11 : Logic  Operator=OR  AllPortsSameDT=off  OutDataTypeStr=boolean
  Compare To Constant5 : simulink/Logic and Bit Operations/Compare To Constant  relop===  const=0  OutDataTypeStr=boolean
  Constant : Constant  OutDataTypeStr=uint8
  Constant1 : Constant  Value=2  OutDataTypeStr=uint8
  Constant10 : Constant  Value=5  OutDataTypeStr=uint8
  Constant2 : Constant  Value=3  OutDataTypeStr=uint8
  Constant3 : Constant  Value=4  OutDataTypeStr=uint8
  Constant4 : Constant  Value=5  OutDataTypeStr=uint8
  Constant5 : Constant  Value=7  OutDataTypeStr=uint8
  Constant6 : Constant  OutDataTypeStr=uint8
  Constant7 : Constant  Value=2  OutDataTypeStr=uint8
  Constant8 : Constant  Value=3  OutDataTypeStr=uint8
  Constant9 : Constant  Value=4  OutDataTypeStr=uint8
  Data Type Conversion{1..9,13} (10 alike) : DataTypeConversion  OutDataTypeStr=uint8
  Detect Change1 : simulink/Logic and Bit Operations/Detect Change  vinit=0  OutDataTypeStr=boolean
  Detect Change7 : simulink/Logic and Bit Operations/Detect Change  vinit=0  OutDataTypeStr=boolean
  Logical Operator1 : Logic  AllPortsSameDT=off  OutDataTypeStr=boolean
  Multiport Switch : MultiPortSwitch  Inputs=7  DataPortForDefault=Additional data port  DiagnosticForDefault=None
  NOT : Logic  Operator=NOT  IconShape=distinctive  AllPortsSameDT=off  OutDataTypeStr=boolean
  OR{,1..4} (5 alike) : Logic  Operator=OR  AllPortsSameDT=off  OutDataTypeStr=boolean
  Relational Operator{,1..5,7..11} (11 alike) : RelationalOperator  Operator===  OutDataTypeStr=boolean  RndMeth=Simplest
  Switch{,1..3,5,7..8,12..13} (9 alike) : Switch  Criteria=u2 ~= 0
  Switch{4,6,9..11} (5 alike) : Switch  Criteria=u2 > Threshold
  Unit Delay{1..13} (13 alike) : UnitDelay  SampleTime=-1  HasFrameUpgradeWarning=on
  Setting : Outport
  Set1 : Outport  Port=2
  Set2 : Outport  Port=3
  Set3 : Outport  Port=4
  Set4 : Outport  Port=5
  Set5 : Outport  Port=6
  Set7 : Outport  Port=7
  wires:
  [Loadbar] -> Logical Operator1/2
  Data Type Conversion9/1 -> Relational Operator4/2
  Unit Delay12/1 -> OR4/1
  OR4/1 -> Switch13/2
  Constant10/1 -> Data Type Conversion8/1
  [UpdateReq] -> Relational Operator11/1
  Data Type Conversion8/1 -> Relational Operator11/2
  Relational Operator11/1 -> OR4/2
  Data Type Conversion7/1 -> Relational Operator3/2
  Constant3/1 -> Data Type Conversion7/1
  OR3/1 -> Switch7/2
  Unit Delay11/1 -> OR3/1
  Relational Operator10/1 -> OR3/2
  Data Type Conversion6/1 -> Relational Operator10/2
  [UpdateReq] -> Relational Operator10/1
  Constant9/1 -> Data Type Conversion6/1
  Data Type Conversion5/1 -> Relational Operator2/2
  Constant2/1 -> Data Type Conversion5/1
  OR2/1 -> Switch5/2
  Unit Delay10/1 -> OR2/1
  Constant8/1 -> Data Type Conversion4/1
  [UpdateReq] -> Relational Operator9/1
  Data Type Conversion4/1 -> Relational Operator9/2
  Relational Operator9/1 -> OR2/2
  Data Type Conversion3/1 -> Relational Operator1/2
  Unit Delay9/1 -> OR1/1
  OR1/1 -> Switch3/2
  Relational Operator8/1 -> OR1/2
  Data Type Conversion2/1 -> Relational Operator8/2
  [UpdateReq] -> Relational Operator8/1
  Constant7/1 -> Data Type Conversion2/1
  Data Type Conversion1/1 -> Relational Operator/2
  Unit Delay6/1 -> OR/1
  OR/1 -> Switch2/2
  Constant6/1 -> Data Type Conversion13/1
  [UpdateReq] -> Relational Operator7/1
  Data Type Conversion13/1 -> Relational Operator7/2
  Relational Operator7/1 -> OR/2
  UpdateReq/1 -> [UpdateReq]
  Unit Delay13/1 -> Switch12/2
  Unit Delay5/1 -> Switch12/3
  Unit Delay4/1 -> Switch13/3
  Unit Delay3/1 -> Switch7/3
  Unit Delay8/1 -> Switch5/3
  Unit Delay2/1 -> Switch3/3
  Unit Delay7/1 -> Switch2/3
  Unit Delay1/1 -> Setting/1, [Set], Switch1/1
  Switch/1 -> Unit Delay1/1
  Loadbar/1 -> Compare To Constant5/1, [Loadbar]
  UserNow/1 -> Detect Change7/1, [UserNow], Multiport Switch/1
  Compare To Constant5/1 -> AND11/1
  AND11/1 -> NOT/1
  [Set7] -> Set7/1
  [Set5] -> Set5/1
  [Set4] -> Set4/1
  [Set3] -> Set3/1
  [Set2] -> Set2/1
  [Set1] -> Set1/1
  Switch1/1 -> Switch/3
  Logical Operator1/1 -> Switch/2
  Multiport Switch/1 -> Switch1/3
  SettingIN/1 -> Switch/1, Detect Change1/1
  Detect Change1/1 -> Logical Operator1/1
  Switch6/1 -> Unit Delay8/1, [Set3]
  Switch2/1 -> Switch8/1
  Switch12/1 -> Switch11/1
  Switch5/1 -> Switch6/1
  Switch13/1 -> Switch10/1
  [Set] -> Switch5/1
  EEP_Set1/1 -> Switch8/3
  Switch9/1 -> Unit Delay3/1, [Set4]
  EEP_Set7/1 -> Switch11/3
  [Loadbar] -> Switch9/2
  [Set] -> Switch12/1
  Relational Operator/1 -> Unit Delay6/1
  [Set] -> Switch13/1
  [Set] -> Switch3/1
  [Loadbar] -> Switch10/2
  Constant/1 -> Data Type Conversion1/1
  [Loadbar] -> Switch6/2
  [Loadbar] -> Switch11/2
  EEP_Set5/1 -> Switch10/3
  EEP_Set2/1 -> Switch4/3
  [UserNow] -> Relational Operator/1
  Switch4/1 -> Unit Delay2/1, [Set2]
  [Loadbar] -> Switch4/2
  [Set] -> Switch7/1
  EEP_Set4/1 -> Switch9/3
  Switch11/1 -> Unit Delay5/1, [Set7]
  EEP_Set3/1 -> Switch6/3
  [Loadbar] -> Switch8/2
  [UserNow] -> Relational Operator1/1
  Constant1/1 -> Data Type Conversion3/1
  Relational Operator1/1 -> Unit Delay9/1
  [UserNow] -> Relational Operator2/1
  Relational Operator2/1 -> Unit Delay10/1
  [UserNow] -> Relational Operator3/1
  Relational Operator3/1 -> Unit Delay11/1
  [UserNow] -> Relational Operator4/1
  Constant4/1 -> Data Type Conversion9/1
  Relational Operator4/1 -> Unit Delay12/1
  [UserNow] -> Relational Operator5/1
  Constant5/1 -> Relational Operator5/2
  Relational Operator5/1 -> Unit Delay13/1
  Switch3/1 -> Switch4/1
  Detect Change7/1 -> AND11/2
  Switch7/1 -> Switch9/1
  Switch10/1 -> Unit Delay4/1, [Set5]
  Switch8/1 -> Unit Delay7/1, [Set1]
  NOT/1 -> Switch1/2
  [Set] -> Switch2/1
  [Set1] -> Multiport Switch/2
  [Set2] -> Multiport Switch/3
  [Set3] -> Multiport Switch/4
  [Set4] -> Multiport Switch/5
  [Set5] -> Multiport Switch/6
  [Set7] -> Multiport Switch/8
  Default/1 -> Multiport Switch/9, Multiport Switch/7

== system thc/THC/ThermalControl/AC/VALUE_TYPE_FDCTHCCREVentZSta ==
  UserNow : Inport
  Loadbar : Inport  Port=2
  UpdateReq : Inport  Port=3
  SettingIN : Inport  Port=4
  EEP_Set1 : Inport  Port=5
  EEP_Set2 : Inport  Port=6
  EEP_Set3 : Inport  Port=7
  EEP_Set4 : Inport  Port=8
  EEP_Set5 : Inport  Port=9
  EEP_Set7 : Inport  Port=10
  Default : Inport  Port=11
  AND11 : Logic  Operator=OR  AllPortsSameDT=off  OutDataTypeStr=boolean
  Compare To Constant5 : simulink/Logic and Bit Operations/Compare To Constant  relop===  const=0  OutDataTypeStr=boolean
  Constant : Constant  OutDataTypeStr=uint8
  Constant1 : Constant  Value=2  OutDataTypeStr=uint8
  Constant10 : Constant  Value=5  OutDataTypeStr=uint8
  Constant2 : Constant  Value=3  OutDataTypeStr=uint8
  Constant3 : Constant  Value=4  OutDataTypeStr=uint8
  Constant4 : Constant  Value=5  OutDataTypeStr=uint8
  Constant5 : Constant  Value=7  OutDataTypeStr=uint8
  Constant6 : Constant  OutDataTypeStr=uint8
  Constant7 : Constant  Value=2  OutDataTypeStr=uint8
  Constant8 : Constant  Value=3  OutDataTypeStr=uint8
  Constant9 : Constant  Value=4  OutDataTypeStr=uint8
  Data Type Conversion{1..9,13} (10 alike) : DataTypeConversion  OutDataTypeStr=uint8
  Detect Change1 : simulink/Logic and Bit Operations/Detect Change  vinit=0  OutDataTypeStr=boolean
  Detect Change7 : simulink/Logic and Bit Operations/Detect Change  vinit=0  OutDataTypeStr=boolean
  Logical Operator1 : Logic  AllPortsSameDT=off  OutDataTypeStr=boolean
  Multiport Switch : MultiPortSwitch  Inputs=7  DataPortForDefault=Additional data port  DiagnosticForDefault=None
  NOT : Logic  Operator=NOT  IconShape=distinctive  AllPortsSameDT=off  OutDataTypeStr=boolean
  OR{,1..4} (5 alike) : Logic  Operator=OR  AllPortsSameDT=off  OutDataTypeStr=boolean
  Relational Operator{,1..5,7..11} (11 alike) : RelationalOperator  Operator===  OutDataTypeStr=boolean  RndMeth=Simplest
  Switch{,1..3,5,7..8,12..13} (9 alike) : Switch  Criteria=u2 ~= 0
  Switch{4,6,9..11} (5 alike) : Switch  Criteria=u2 > Threshold
  Unit Delay{1..13} (13 alike) : UnitDelay  SampleTime=-1  HasFrameUpgradeWarning=on
  Setting : Outport
  Set1 : Outport  Port=2
  Set2 : Outport  Port=3
  Set3 : Outport  Port=4
  Set4 : Outport  Port=5
  Set5 : Outport  Port=6
  Set7 : Outport  Port=7
  wires:
  [Loadbar] -> Logical Operator1/2
  Data Type Conversion9/1 -> Relational Operator4/2
  Unit Delay12/1 -> OR4/1
  OR4/1 -> Switch13/2
  Constant10/1 -> Data Type Conversion8/1
  [UpdateReq] -> Relational Operator11/1
  Data Type Conversion8/1 -> Relational Operator11/2
  Relational Operator11/1 -> OR4/2
  Data Type Conversion7/1 -> Relational Operator3/2
  Constant3/1 -> Data Type Conversion7/1
  OR3/1 -> Switch7/2
  Unit Delay11/1 -> OR3/1
  Relational Operator10/1 -> OR3/2
  Data Type Conversion6/1 -> Relational Operator10/2
  [UpdateReq] -> Relational Operator10/1
  Constant9/1 -> Data Type Conversion6/1
  Data Type Conversion5/1 -> Relational Operator2/2
  Constant2/1 -> Data Type Conversion5/1
  OR2/1 -> Switch5/2
  Unit Delay10/1 -> OR2/1
  Constant8/1 -> Data Type Conversion4/1
  [UpdateReq] -> Relational Operator9/1
  Data Type Conversion4/1 -> Relational Operator9/2
  Relational Operator9/1 -> OR2/2
  Data Type Conversion3/1 -> Relational Operator1/2
  Unit Delay9/1 -> OR1/1
  OR1/1 -> Switch3/2
  Relational Operator8/1 -> OR1/2
  Data Type Conversion2/1 -> Relational Operator8/2
  [UpdateReq] -> Relational Operator8/1
  Constant7/1 -> Data Type Conversion2/1
  Data Type Conversion1/1 -> Relational Operator/2
  Unit Delay6/1 -> OR/1
  OR/1 -> Switch2/2
  Constant6/1 -> Data Type Conversion13/1
  [UpdateReq] -> Relational Operator7/1
  Data Type Conversion13/1 -> Relational Operator7/2
  Relational Operator7/1 -> OR/2
  UpdateReq/1 -> [UpdateReq]
  Unit Delay13/1 -> Switch12/2
  Unit Delay5/1 -> Switch12/3
  Unit Delay4/1 -> Switch13/3
  Unit Delay3/1 -> Switch7/3
  Unit Delay8/1 -> Switch5/3
  Unit Delay2/1 -> Switch3/3
  Unit Delay7/1 -> Switch2/3
  Unit Delay1/1 -> Setting/1, [Set], Switch1/1
  Switch/1 -> Unit Delay1/1
  Loadbar/1 -> Compare To Constant5/1, [Loadbar]
  UserNow/1 -> Detect Change7/1, [UserNow], Multiport Switch/1
  Compare To Constant5/1 -> AND11/1
  AND11/1 -> NOT/1
  [Set7] -> Set7/1
  [Set5] -> Set5/1
  [Set4] -> Set4/1
  [Set3] -> Set3/1
  [Set2] -> Set2/1
  [Set1] -> Set1/1
  Switch1/1 -> Switch/3
  Logical Operator1/1 -> Switch/2
  Multiport Switch/1 -> Switch1/3
  SettingIN/1 -> Switch/1, Detect Change1/1
  Detect Change1/1 -> Logical Operator1/1
  Switch6/1 -> Unit Delay8/1, [Set3]
  Switch2/1 -> Switch8/1
  Switch12/1 -> Switch11/1
  Switch5/1 -> Switch6/1
  Switch13/1 -> Switch10/1
  [Set] -> Switch5/1
  EEP_Set1/1 -> Switch8/3
  Switch9/1 -> Unit Delay3/1, [Set4]
  EEP_Set7/1 -> Switch11/3
  [Loadbar] -> Switch9/2
  [Set] -> Switch12/1
  Relational Operator/1 -> Unit Delay6/1
  [Set] -> Switch13/1
  [Set] -> Switch3/1
  [Loadbar] -> Switch10/2
  Constant/1 -> Data Type Conversion1/1
  [Loadbar] -> Switch6/2
  [Loadbar] -> Switch11/2
  EEP_Set5/1 -> Switch10/3
  EEP_Set2/1 -> Switch4/3
  [UserNow] -> Relational Operator/1
  Switch4/1 -> Unit Delay2/1, [Set2]
  [Loadbar] -> Switch4/2
  [Set] -> Switch7/1
  EEP_Set4/1 -> Switch9/3
  Switch11/1 -> Unit Delay5/1, [Set7]
  EEP_Set3/1 -> Switch6/3
  [Loadbar] -> Switch8/2
  [UserNow] -> Relational Operator1/1
  Constant1/1 -> Data Type Conversion3/1
  Relational Operator1/1 -> Unit Delay9/1
  [UserNow] -> Relational Operator2/1
  Relational Operator2/1 -> Unit Delay10/1
  [UserNow] -> Relational Operator3/1
  Relational Operator3/1 -> Unit Delay11/1
  [UserNow] -> Relational Operator4/1
  Constant4/1 -> Data Type Conversion9/1
  Relational Operator4/1 -> Unit Delay12/1
  [UserNow] -> Relational Operator5/1
  Constant5/1 -> Relational Operator5/2
  Relational Operator5/1 -> Unit Delay13/1
  Switch3/1 -> Switch4/1
  Detect Change7/1 -> AND11/2
  Switch7/1 -> Switch9/1
  Switch10/1 -> Unit Delay4/1, [Set5]
  Switch8/1 -> Unit Delay7/1, [Set1]
  NOT/1 -> Switch1/2
  [Set] -> Switch2/1
  [Set1] -> Multiport Switch/2
  [Set2] -> Multiport Switch/3
  [Set3] -> Multiport Switch/4
  [Set4] -> Multiport Switch/5
  [Set5] -> Multiport Switch/6
  [Set7] -> Multiport Switch/8
  Default/1 -> Multiport Switch/9, Multiport Switch/7
